simulink model "single_track"  (R2017a)
settings: Solver=VariableStepAuto  StartTime=0.0  StopTime=10.0  RelTol=1e-3
values from neighbouring files (symbols this model uses):
  SIM_Tsolver = 1e-4    (= 0.0001)    [test_beta_estimator_init.m]
undefined symbols (not defined in the file or in its folder): Clock_, clock_publishing_period, measure_publishing_period, param, singleTrack_equation, Theta, X, Y
libraries: robotlib x6
settings Model: Creator=bascetta  LastModifiedBy=bascetta

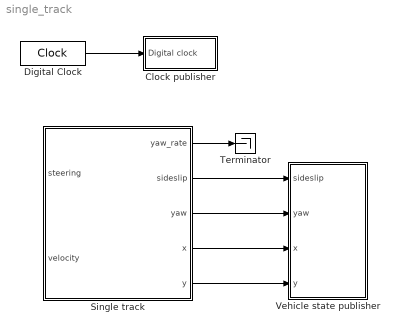
== system single_track ==
  Clock publisher : Subsystem
  Digital Clock : DigitalClock  SampleTime=SIM_Tsolver
  Single track : Subsystem  mask{param=param}
      mask prompts: param "Vehicle parameter vector"
  Terminator : Terminator
  Vehicle state publisher : Subsystem
  wires:
  Single track/4(x) -> Vehicle state publisher/3(x)
  Single track/5(y) -> Vehicle state publisher/4(y)
  Single track/3(yaw) -> Vehicle state publisher/2(yaw)
  Single track/2(sideslip) -> Vehicle state publisher/1(sideslip)
  Single track/1(yaw_rate) -> Terminator/1
  Digital Clock/1 -> Clock publisher/1(Digital clock)

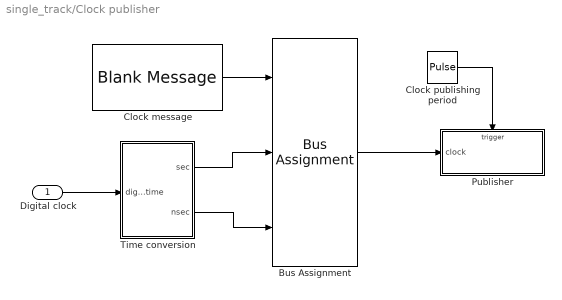
== system single_track/Clock publisher ==
  Digital clock : Inport
  Bus Assignment : BusAssignment  DialogController=Simulink.DDGSource_BusAssignment  AssignedSignals=Clock_.Sec,Clock_.Nsec
  Clock message : robotlib/Blank Message  SourceLibraryInfo=This block requires Robotics System Toolbox  messageType=rosgraph_msgs/Clock  SampleTime=inf
      settings: SourceProductBaseCode=RO
  Clock publishing period : DiscretePulseGenerator  PulseType=Time based  Period=clock_publishing_period  PulseWidth=50
  Publisher : Subsystem  TreatAsAtomicUnit=on
  Time conversion : MATLAB Function  TreatAsAtomicUnit=on
  wires:
  Clock message/1 -> Bus Assignment/1
  Bus Assignment/1 -> Publisher/1(clock)
  Time conversion/1(sec) -> Bus Assignment/2
  Time conversion/2(nsec) -> Bus Assignment/3
  Digital clock/1 -> Time conversion/1(digital_time)
  Clock publishing period/1 -> Publisher/Trigger

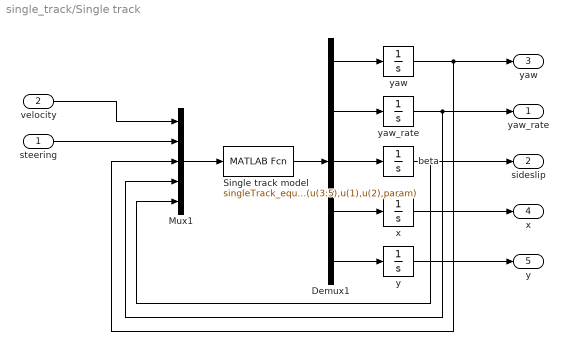
== system single_track/Single track ==
  steering : Inport
  velocity : Inport  Port=2
  Demux1 : Demux  Outputs=5
  Mux1 : Mux  Inputs=5
  Single track model : MATLABFcn  MATLABFcn=singleTrack_equation(u(3:5),u(1),u(2),param)  OutputDimensions=5
  "beta " : Integrator
  "x " : Integrator
  "y " : Integrator
  "yaw " : Integrator
  "yaw_rate " : Integrator
  yaw_rate : Outport
  sideslip : Outport  Port=2
  yaw : Outport  Port=3
  x : Outport  Port=4
  y : Outport  Port=5
  wires:
  Single track model/1 -> Demux1/1
  "yaw_rate "/1 -> Mux1/4, yaw_rate/1
  Mux1/1 -> Single track model/1
  "beta "/1 -> Mux1/5, sideslip/1
  "yaw "/1 -> Mux1/3, yaw/1
  Demux1/1 -> "yaw "/1
  Demux1/2 -> "yaw_rate "/1
  Demux1/3 -> "beta "/1
  Demux1/4 -> "x "/1
  Demux1/5 -> "y "/1
  "x "/1 -> x/1
  "y "/1 -> y/1
  steering/1 -> Mux1/2
  velocity/1 -> Mux1/1

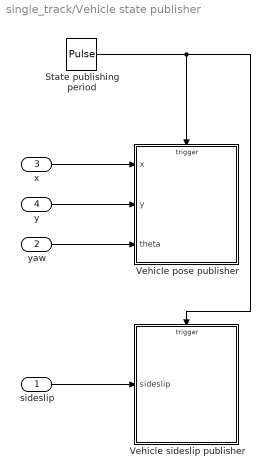
== system single_track/Vehicle state publisher ==
  sideslip : Inport
  yaw : Inport  Port=2
  x : Inport  Port=3
  y : Inport  Port=4
  State publishing period : DiscretePulseGenerator  PulseType=Time based  Period=measure_publishing_period  PulseWidth=50
  Vehicle pose publisher : Subsystem  TreatAsAtomicUnit=on
  Vehicle sideslip publisher : Subsystem  TreatAsAtomicUnit=on
  wires:
  State publishing period/1 -> Vehicle sideslip publisher/Trigger, Vehicle pose publisher/Trigger
  x/1 -> Vehicle pose publisher/1(x)
  y/1 -> Vehicle pose publisher/2(y)
  yaw/1 -> Vehicle pose publisher/3(theta)
  sideslip/1 -> Vehicle sideslip publisher/1(sideslip)

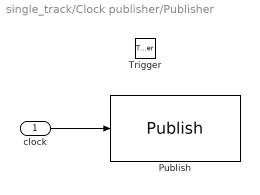
== system single_track/Clock publisher/Publisher ==
  clock : Inport
  Trigger : TriggerPort  VariantControl=Variant
  Publish : robotlib/Publish  SourceLibraryInfo=This block requires Robotics System Toolbox  topicSource=Specify your own  topic=/clock  messageType=rosgraph_msgs/Clock  messageQueueLength=1
      settings: SourceProductBaseCode=RO
  wires:
  clock/1 -> Publish/1

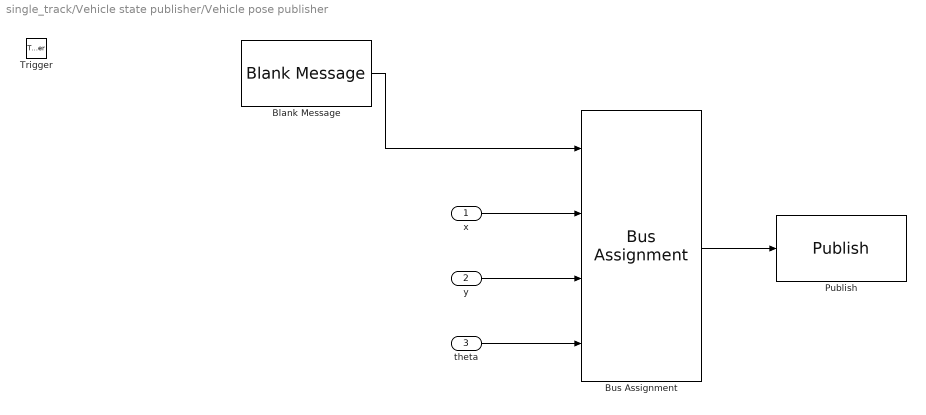
== system single_track/Vehicle state publisher/Vehicle pose publisher ==
  x : Inport
  y : Inport  Port=2
  theta : Inport  Port=3
  Trigger : TriggerPort  VariantControl=Variant
  Blank Message : robotlib/Blank Message  SourceLibraryInfo=This block requires Robotics System Toolbox  messageType=geometry_msgs/Pose2D  SampleTime=inf
      settings: SourceProductBaseCode=RO
  Bus Assignment : BusAssignment  DialogController=Simulink.DDGSource_BusAssignment  AssignedSignals=X,Y,Theta
  Publish : robotlib/Publish  SourceLibraryInfo=This block requires Robotics System Toolbox  topicSource=Select from ROS network  topic=/vehiclePose  messageType=geometry_msgs/Pose2D  messageQueueLength=1
      settings: SourceProductBaseCode=RO
  wires:
  Blank Message/1 -> Bus Assignment/1
  Bus Assignment/1 -> Publish/1
  theta/1 -> Bus Assignment/4
  y/1 -> Bus Assignment/3
  x/1 -> Bus Assignment/2

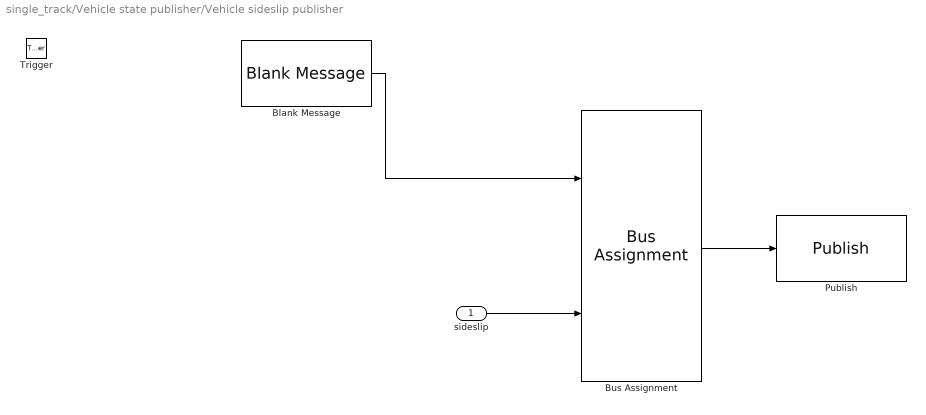
== system single_track/Vehicle state publisher/Vehicle sideslip publisher ==
  sideslip : Inport
  Trigger : TriggerPort  VariantControl=Variant
  Blank Message : robotlib/Blank Message  SourceLibraryInfo=This block requires Robotics System Toolbox  messageType=std_msgs/Float64  SampleTime=inf
      settings: SourceProductBaseCode=RO
  Bus Assignment : BusAssignment  DialogController=Simulink.DDGSource_BusAssignment  AssignedSignals=Data
  Publish : robotlib/Publish  SourceLibraryInfo=This block requires Robotics System Toolbox  topicSource=Specify your own  topic=/vehicleSideslip  messageType=std_msgs/Float64  messageQueueLength=1
      settings: SourceProductBaseCode=RO
  wires:
  Blank Message/1 -> Bus Assignment/1
  Bus Assignment/1 -> Publish/1
  sideslip/1 -> Bus Assignment/2

== matlab function single_track/Clock publisher/Time conversion ==
  data: digital_time input; sec output; nsec output
function [sec,nsec] = time2rosclock(digital_time)

sec = floor(digital_time);
nsec = round((digital_time-sec)*1.0e+9);
